simulink subsystem "Drag_Force"  (R2023a)
settings: Solver=VariableStepAuto  StartTime=0.0  StopTime=10.0  RelTol=1e-3
undefined symbols (not defined in the file): angular, linear
libraries: dspstat3 x6, ros2lib x4

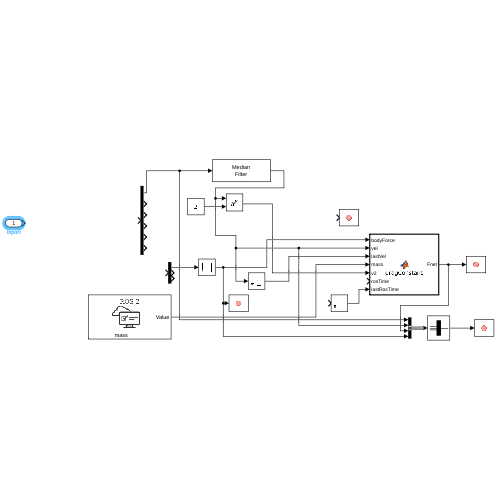
[thumbnail: Simulink's stored preview of the top-level diagram]
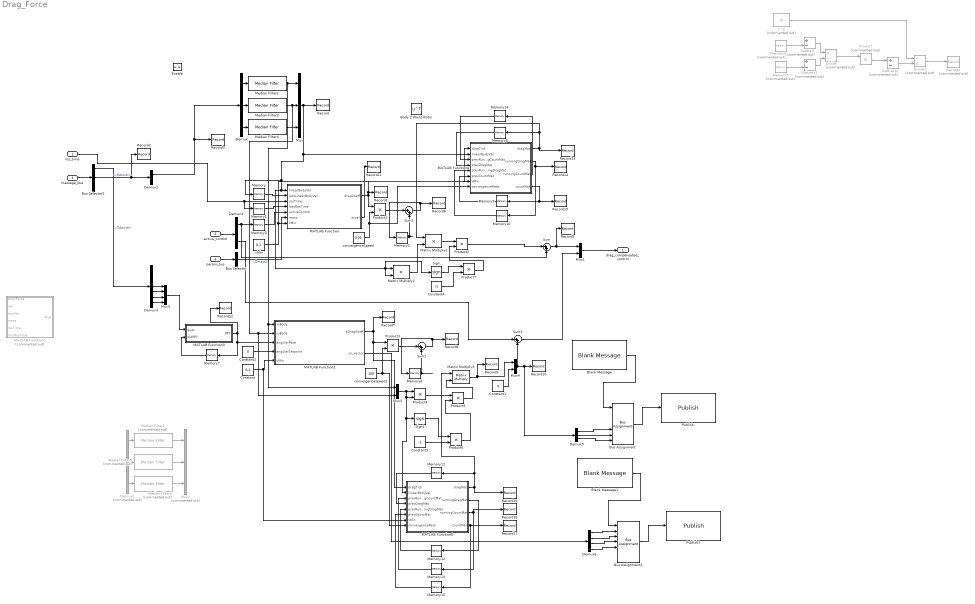
== system Drag_Force ==
  ros_time : Inport
  active_control : Inport  Port=2
  message_bus : Inport  Port=3
  param_bus : Inport  Port=4
  Enable : EnablePort
  Blank Message : ros2lib/Blank Message  messageClass=Message  entityType=geometry_msgs/Twist  messageType=geometry_msgs/Twist  SampleTime=inf
  Blank Message1 : ros2lib/Blank Message  messageClass=Message  entityType=geometry_msgs/Twist  messageType=geometry_msgs/Twist  SampleTime=inf
  Body 2 World Rotm : Math  Operator=transpose
  Bus Assignment : BusAssignment  AssignedSignals=linear.x,linear.y,linear.z,angular.x,angular.y,angular.z
  Bus Assignment1 : BusAssignment  AssignedSignals=linear.x,linear.y,linear.z,angular.x,angular.y,angular.z
  Bus Selector : BusSelector  OutputSignals=Dmass
  Bus Selector2 : BusSelector  OutputSignals=current_state.DApose,current_state.DAtwist,desired_pose.DAdesired_pose
  Constant : Constant  Value=0.2
  Constant1 : Constant  Value=0
  Constant2 : Constant  Value=0
  Constant3 : Constant  Value=-1
  Constant4 : Constant  Value=-1
  Demux : Demux  Outputs=3
  Demux1 : Demux  Outputs=2
  Demux2 : Demux  Commented=on  Outputs=3
  Demux3 : Demux  Outputs=7
  Demux4 : Demux  Outputs=2
  Demux5 : Demux  Outputs=3
  Demux6 : Demux
  Divide : Product  Commented=on  Inputs=*/
  Divide1 : Product  Commented=on  Inputs=/*
  MATLAB Function : MATLAB Function  TreatAsAtomicUnit=on
  MATLAB Function1 : MATLAB Function  Commented=on  TreatAsAtomicUnit=on
  MATLAB Function2 : MATLAB Function  TreatAsAtomicUnit=on
  MATLAB Function3 : MATLAB Function  TreatAsAtomicUnit=on
  MATLAB Function4 : MATLAB Function  TreatAsAtomicUnit=on
  MATLAB Function6 : MATLAB Function  TreatAsAtomicUnit=on
  Matrix Multiply1 : Product
  Matrix Multiply2 : Product
  Matrix Multiply3 : Product  Multiplication=Matrix(*)
  Median Filter1 : dspstat3/Median Filter  Commented=on  WindowLength=20  SimulateUsing=Interpreted execution
  Median Filter2 : dspstat3/Median Filter  WindowLength=20  SimulateUsing=Interpreted execution
  Median Filter3 : dspstat3/Median Filter  WindowLength=20  SimulateUsing=Interpreted execution
  Median Filter4 : dspstat3/Median Filter  WindowLength=20  SimulateUsing=Interpreted execution
  Median Filter5 : dspstat3/Median Filter  Commented=on  WindowLength=20  SimulateUsing=Interpreted execution
  Median Filter6 : dspstat3/Median Filter  Commented=on  WindowLength=20  SimulateUsing=Interpreted execution
  Memory{,1..3,6,8..15} (13 alike) : Memory
  Memory4 : Memory  Commented=on
  Memory5 : Memory  Commented=on
  Memory7 : Memory  InitialCondition=[0, 0, 0]
  Mux : Mux  Inputs=3
  Mux1 : Mux  Inputs=2
  Mux2 : Mux  Commented=on  Inputs=3
  Mux3 : Mux  Inputs=2
  Mux4 : Mux  Inputs=2
  Mux5 : Mux
  Product : Product  Commented=on
  Product{1..7} (7 alike) : Product
  Publish : ros2lib/Publish  topicSource=Specify your own  topic=/drag_4ce  messageType=geometry_msgs/Twist  QOSHistory=Keep last  QOSDepth=1  QOSReliability=Reliable  QOSDurability=Volatile
  Publish1 : ros2lib/Publish  topicSource=Specify your own  topic=/learned_matrix  messageType=geometry_msgs/Twist  QOSHistory=Keep last  QOSDepth=1  QOSReliability=Reliable  QOSDurability=Volatile
  Record{,1..3,5..18} (18 alike) : Record  FileSettingsInternal="{\"entries\":[{\"content\":{\"excelSettings\":{\"content\":{},\"type\":\"Streamout.ExcelSettings\"}},\"type\":\"Streamout.FileSettingStorage\",\"uuid\":\"\"}],\"packageUris\":[\"http:\\/\\/schema.mathworks.com\\/mf0\\/streamout_blocks\\/R2020a\"],\"version\":\"1.0\"}"  SignalsInternal="{\"entries\":[{\"content\":{},\"type\":\"RecordBlkView.InputSignals\",\"uuid\":\"\"}],\"packageUris\":[\"http:\\/\\/schema.mathworks.com\\/mf0\\/streamout_blocks\\/R2020a\"],\"version\":\"1.0\"}"  VisualizationBindings="{\"sparklinesplugin\":{\"info\":[{\"bindingParametersList\":[],\"subplotID\":1}]}}"
  Record4 : Record  Commented=on  FileSettingsInternal="{\"entries\":[{\"content\":{\"excelSettings\":{\"content\":{},\"type\":\"Streamout.ExcelSettings\"}},\"type\":\"Streamout.FileSettingStorage\",\"uuid\":\"\"}],\"packageUris\":[\"http:\\/\\/schema.mathworks.com\\/mf0\\/streamout_blocks\\/R2020a\"],\"version\":\"1.0\"}"  SignalsInternal="{\"entries\":[{\"content\":{},\"type\":\"RecordBlkView.InputSignals\",\"uuid\":\"\"}],\"packageUris\":[\"http:\\/\\/schema.mathworks.com\\/mf0\\/streamout_blocks\\/R2020a\"],\"version\":\"1.0\"}"  VisualizationBindings="{\"sparklinesplugin\":{\"info\":[{\"bindingParametersList\":[],\"subplotID\":1}]}}"
  Sign : Signum
  Sign1 : Signum
  Subtract : Sum  Commented=on  Inputs=+-
  Subtract1 : Sum  Commented=on  Inputs=+-
  Subtract2 : Sum  Commented=on  Inputs=+-
  Sum{,1..3} (4 alike) : Sum  Inputs=|++
  convergenceSpeed : Constant  Value=0.05
  convergenceSpeed1 : Constant  Value=100
  vMin : Constant  Value=0.1
  v^2 : Product  Commented=on
  drag_compensated_control : Outport
  wires:
  Demux4/1 -> Memory3/1, Sum/2
  message_bus/1 -> Bus Selector2/1
  Bus Selector2/2 -> Record2/1, Demux1/1  "<DAtwist>"
  active_control/1 -> Demux4/1
  Memory4/1 -> Subtract/2
  Memory5/1 -> Subtract1/2
  Subtract/1 -> Divide/1
  Subtract1/1 -> Divide/2
  param_bus/1 -> Bus Selector/1
  Divide/1 -> Product/1
  Product/1 -> Subtract2/1
  Subtract2/1 -> Divide1/2
  v^2/1 -> Divide1/1
  Divide1/1 -> Record4/1
  Memory/1 -> MATLAB Function/2(lastLinearBodyVel)
  ros_time/1 -> MATLAB Function/3(rosTime), Memory1/1
  Memory1/1 -> MATLAB Function/4(lastRosTime)
  Bus Selector/1 -> MATLAB Function/6(mass)  "<Dmass>"
  Memory3/1 -> MATLAB Function/5(activeControl)
  vMin/1 -> MATLAB Function/7(vMin), MATLAB Function4/7(vMin)
  MATLAB Function/1(dragCoeff) -> Product1/1, Record1/1, MATLAB Function4/1(dragTick)
  Demux/1 -> Median Filter2/1
  Demux/2 -> Median Filter3/1
  Demux/3 -> Median Filter4/1
  Median Filter2/1 -> Mux/1, MATLAB Function2/1(vxBody), Mux3/1
  Median Filter3/1 -> Mux/2, Mux3/2, MATLAB Function2/2(vyBody)
  Median Filter4/1 -> Mux/3
  Mux/1 -> Record/1, Matrix Multiply2/1, Matrix Multiply2/2, Sign/1, MATLAB Function/1(linearBodyVel), Memory/1, MATLAB Function4/2(linearBodyVel)
  Memory2/1 -> Sum1/2
  Sum1/1 -> Memory2/1, Record6/1
  convergenceSpeed/1 -> Product1/2, MATLAB Function4/8(convergenceRate)
  Product1/1 -> Sum1/1
  Sum/1 -> Record5/1, Mux1/1
  Matrix Multiply2/1 -> Matrix Multiply1/2
  Mux1/1 -> drag_compensated_control/1
  Demux4/2 -> Sum3/1
  Sign/1 -> Product7/1
  Matrix Multiply1/1 -> Product2/1
  Product2/1 -> Sum/1
  Constant/1 -> MATLAB Function2/5(vMin), MATLAB Function6/7(vMin)
  Constant2/1 -> MATLAB Function2/4(angularSetpoint)
  MATLAB Function2/1(aDragCoeff) -> Record7/1, Product3/1, MATLAB Function6/1(dragTick)
  Memory6/1 -> Sum2/2
  Product3/1 -> Sum2/1
  convergenceSpeed1/1 -> Product3/2, MATLAB Function6/8(convergenceRate)
  Demux2/2 -> Median Filter5/1
  Median Filter5/1 -> Mux2/2
  Median Filter6/1 -> Mux2/3
  Median Filter1/1 -> Mux2/1
  Demux2/3 -> Median Filter6/1
  Demux2/1 -> Median Filter1/1
  Mux3/1 -> Product4/1, Product4/2, Sign1/1, MATLAB Function6/2(linearBodyVel)
  Product4/1 -> Product5/1
  Matrix Multiply3/1 -> Record9/1, Mux4/1
  Sum3/1 -> Mux1/2
  Mux4/1 -> Sum3/2, Record10/1, Demux5/1
  Constant1/1 -> Mux4/2
  Sign1/1 -> Product6/1
  Product5/1 -> Matrix Multiply3/2
  Bus Selector2/1 -> Demux3/1  "<DApose>"
  Demux3/4 -> Mux5/1
  Demux3/5 -> Mux5/2
  Demux3/6 -> Mux5/3
  Demux3/7 -> Mux5/4
  Mux5/1 -> MATLAB Function3/1(quat)
  Memory7/1 -> MATLAB Function3/2(oldRPY)
  MATLAB Function3/1(RPY) -> Record12/1, Memory7/1, MATLAB Function2/3(angularPose)
  Bus Assignment/1 -> Publish/1
  Blank Message/1 -> Bus Assignment/1
  Demux5/1 -> Bus Assignment/5
  Demux5/2 -> Bus Assignment/6
  Demux5/3 -> Bus Assignment/7
  Bus Assignment1/1 -> Publish1/1
  Blank Message1/1 -> Bus Assignment1/1
  Sum2/1 -> Memory6/1, Record8/1
  MATLAB Function2/2(co_vector) -> Demux6/1
  Demux6/1 -> Bus Assignment1/2
  Demux6/2 -> Bus Assignment1/3
  Demux6/3 -> Bus Assignment1/4
  Demux6/4 -> Bus Assignment1/5
  Constant3/1 -> Product6/2
  Product6/1 -> Product5/2
  MATLAB Function/2(accel) -> Record11/1
  Constant4/1 -> Product7/2
  Product7/1 -> Product2/2
  MATLAB Function4/1(dragMat) -> Memory8/1, Matrix Multiply1/1, Record13/1
  Memory8/1 -> MATLAB Function4/4(prevDragMat)
  Memory9/1 -> MATLAB Function4/6(prevCountMat)
  MATLAB Function4/4(countMat) -> Memory9/1, Record15/1
  MATLAB Function4/2(runningDragMat) -> Memory10/1, Record14/1
  Memory10/1 -> MATLAB Function4/5(prevRunningDragMat)
  MATLAB Function6/1(dragMat) -> Record16/1, Memory11/1, Matrix Multiply3/1
  Memory11/1 -> MATLAB Function6/4(prevDragMat)
  MATLAB Function6/2(runningDragMat) -> Memory12/1
  Memory12/1 -> MATLAB Function6/5(prevRunningDragMat)
  MATLAB Function6/3(runningCountMat) -> Record18/1, Memory13/1
  Memory13/1 -> MATLAB Function6/3(prevRunningCountMat)
  MATLAB Function4/3(runningCountMat) -> Memory14/1
  Memory14/1 -> MATLAB Function4/3(prevRunningCountMat)
  Demux1/1 -> Demux/1, Record3/1
  MATLAB Function6/4(countMat) -> Memory15/1, Record17/1
  Memory15/1 -> MATLAB Function6/6(prevCountMat)

== matlab function Drag_Force/MATLAB Function6 ==
function [dragMat, runningDragMat, runningCountMat, countMat] = fcn(dragTick, linearBodyVel, prevRunningCountMat, prevDragMat, prevRunningDragMat, prevCountMat, vMin, convergenceRate)
dragMat = zeros(2, 2);
countMat = zeros(2, 2);
runningCountMat = zeros(2, 2);
runningDragMat = zeros(2, 2);

for i = 1:size(dragTick, 1)
    for j = 1:2
        if abs(linearBodyVel(i)) < vMin && prevRunningCountMat(i, j) > 0
            prevRunningCountMat(i, j) = prevRunningCountMat(i, j) + 1;
            dragConst = ((prevRunningDragMat(i, j) + dragTick(i, j)) / prevRunningCountMat(i, j)) * convergenceRate;
    
            newCountTotal = prevCountMat(i, j) + prevRunningCountMat(i, j);
            dragMat(i, j) = (prevDragMat(i, j) * prevCountMat(i, j) + dragConst * prevRunningCountMat(i, j)) / newCountTotal;
            countMat(i) = newCountTotal;
    
            runningCountMat(i, j) = 0;
            runningDragMat(i, j) = 0;
        elseif abs(linearBodyVel(i)) > vMin
            runningDragMat(i, j) = dragTick(i, j) + prevRunningDragMat(i, j); 
            runningCountMat(i, j) = prevRunningCountMat(i, j) + 1;
    
            dragMat(i, j) = prevDragMat(i, j);
            countMat(i, j) = prevCountMat(i, j);
        else
            dragMat(i, j) = prevDragMat(i, j);
            countMat(i, j) = prevCountMat(i, j);
        end
    end
end

% function [dragMat, runningDragMat, countMat] = fcn(dragTick, linearBodyVel, prevCountMat, prevDragMat, prevRunningDragMat, vMin, convergenceRate)
% dragMat = zeros(2, 2);
% countMat = zeros(2, 2);
% runningDragMat = zeros(2, 2);
% 
% for i = 1:2
%     for j = 1:2
%         if abs(linearBodyVel(i)) < vMin && prevCountMat(i) > 0
%             dragMat(i, j) = ((prevRunningDragMat(i, j) + dragTick(i, j)) / (prevCountMat(i, j) + 1)) * convergenceRate + prevDragMat(i);
%             countMat(i, j) = 0;
%             runningDragMat(i, j) = 0;
%         elseif abs(linearBodyVel(i)) > vMin
%             runningDragMat(i, j) = dragTick(i, j) + prevRunningDragMat(i, j); 
%             countMat(i, j) = prevCountMat(i, j) + 1;
%             dragMat(i, j) = prevDragMat(i);
%         else
%             dragMat(i, j) = prevDragMat(i, j);
%         end
%     end
% end

== matlab function Drag_Force/MATLAB Function1 ==
function Fnet = dragConstant(bodyForce, vel, lastVel, mass, rosTime, lastRosTime)
Fnet = zeros(1, 3);

for i = 1:size(bodyForce, 1)
    accel = (vel(i) - lastVel(i)) / (rosTime - lastRosTime);
    v2 = vel(i) * vel(i);
    
    if (v2 > 0.1)
        d = ((mass * accel - bodyForce(i)) / (v2));
        fName = "~/drag_data" + i + ".csv";
        file = fopen(fName, "a");
        fprintf(file, "%f\n", d);
        fclose(file);
    end
    
    Fnet(i) = mass * accel;
end

== matlab function Drag_Force/MATLAB Function ==
function [dragCoeff, accel] = linearDragCoeff(linearBodyVel, lastLinearBodyVel, rosTime, lastRosTime, activeControl, mass, vMin)

v2 = linearBodyVel .^ 2;
accel = (linearBodyVel - lastLinearBodyVel) ./ (rosTime - lastRosTime);

dragCoeff = zeros(size(linearBodyVel));
for i = 1:size(linearBodyVel, 1)
    if abs(linearBodyVel(i)) > vMin
        dragCoeff(i) = (mass * accel(i) - activeControl(i)) / v2(i) * sign(linearBodyVel(i));
    end
end

== matlab function Drag_Force/MATLAB Function2 ==
function [aDragCoeff, co_vector] = angularDragCoeff(vxBody, vyBody, angularPose, angularSetpoint, vMin)
aDragCoeff = zeros(2, 2);

for i = 1:2
    if abs(vxBody) > vMin && abs(vyBody) < vMin
        aDragCoeff(i, 1) = ((angularPose(i) - angularSetpoint) / (vxBody * vxBody)) * sign(vxBody);
    elseif abs(vyBody) > vMin
        aDragCoeff(i, 2) = ((angularPose(i) - angularSetpoint) / (vyBody * vyBody)) * sign(vyBody);
    end
end

co_vector = zeros(4,1);

co_vector = [aDragCoeff(1, 1);aDragCoeff(2, 1);aDragCoeff(1, 2);aDragCoeff(2, 2)];

== matlab function Drag_Force/MATLAB Function3 ==
function RPY = unwrapQuat(quat, oldRPY)

eul = rotm2eul(quat2rotm(quat'));

rTmp = unwrap([oldRPY(1), pi - eul(1)]);
pTmp = unwrap([oldRPY(2), -eul(2)]);
yTmp = unwrap([oldRPY(3), eul(3)]);

r = rTmp(2);
p = pTmp(2);
y = yTmp(2);

RPY = [r, p, y];

== matlab function Drag_Force/MATLAB Function4 ==
function [dragMat, runningDragMat, runningCountMat, countMat] = fcn(dragTick, linearBodyVel, prevRunningCountMat, prevDragMat, prevRunningDragMat, prevCountMat, vMin, convergenceRate)
dragMat = zeros(size(linearBodyVel));
countMat = zeros(size(linearBodyVel));
runningCountMat = zeros(size(linearBodyVel));
runningDragMat = zeros(size(linearBodyVel));

for i = 1:size(dragTick, 1)
    if abs(linearBodyVel(i)) < vMin && prevRunningCountMat(i) > 0
        prevRunningCountMat(i) = prevRunningCountMat(i) + 1;
        dragConst = ((prevRunningDragMat(i) + dragTick(i)) / prevRunningCountMat(i)) * convergenceRate;

        newCountTotal = prevCountMat(i) + prevRunningCountMat(i);
        dragMat(i) = (prevDragMat(i) * prevCountMat(i) + dragConst * prevRunningCountMat(i)) / newCountTotal;
        countMat(i) = newCountTotal;

        runningCountMat(i) = 0;
        runningDragMat(i) = 0;
    elseif abs(linearBodyVel(i)) > vMin
        runningDragMat(i) = dragTick(i) + prevRunningDragMat(i); 
        runningCountMat(i) = prevRunningCountMat(i) + 1;

        dragMat(i) = prevDragMat(i);
        countMat(i) = prevCountMat(i);
    else
        dragMat(i) = prevDragMat(i);
        countMat(i) = prevCountMat(i);
    end
end
